simulink model "CEngDsT_DD"  (R2020b)
settings: configuration reference "cs_ert" (kept outside this file)
model workspace (MAT data in the model file):
  CEngDsT_DD_DT = 10
values from neighbouring files (symbols this model uses):
  CEngDsT_MaxCoolTemp = 150.0    [CEngDsT_DD.sldd]
  CEngDsT_MinCoolTemp = -50.0    [CEngDsT_DD.sldd]
  CEngDsT_tiMaxDefDeb_C = 200.0    [CEngDsT_DD.sldd]
  CEngDsT_tiMaxOKDeb_C = 200.0    [CEngDsT_DD.sldd]
  CEngDsT_tiMinDefDeb_C = 200.0    [CEngDsT_DD.sldd]
  CEngDsT_tiMinOKDeb_C = 200.0    [CEngDsT_DD.sldd]
  CEngDsT_tiPhysRngHiDefDeb_C = 200.0    [CEngDsT_DD.sldd]
  CEngDsT_tiPhysRngHiOKDeb_C = 200.0    [CEngDsT_DD.sldd]
  CEngDsT_tiPhysRngLoDefDeb_C = 200.0    [CEngDsT_DD.sldd]
  CEngDsT_tiPhysRngLoOKDeb_C = 200.0    [CEngDsT_DD.sldd]
  CEngDsT_tTransf_CUR : value not decoded    [CEngDsT_DD.sldd]
  CEngDsT_tTransf_CURX : value not decoded    [CEngDsT_DD.sldd]
  CEngDsT_uSRCMax_C = 5000.0    [CEngDsT_DD.sldd]
  CEngDsT_uSRCMin_C = 200.0    [CEngDsT_DD.sldd]
  FM_CEngDsT_SRC_FG_CA : value not decoded    [CEngDsT_DD.sldd]
libraries: sllib x5
settings Model: DataDictionary=CEngDsT_DD.sldd  EnableAccessToBaseWorkspace=off  Creator=zhoutinglin  LastModifiedBy=zhoutinglin
settings ConfigSetRef: SourceName=cs_ert

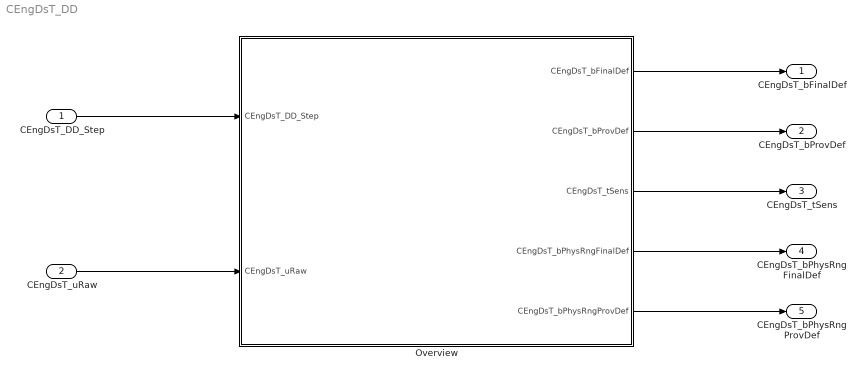
== system CEngDsT_DD ==
  CEngDsT_DD_Step : Inport  OutputFunctionCall=on
  CEngDsT_uRaw : Inport  Description=Raw ADC value of downstream engine coolant temperature sensor signal  Port=2  OutMin=0  OutMax=5000  OutDataTypeStr=Volt_mV2  Unit=mv  PortDimensions=[1 1]
  Overview : Subsystem
  CEngDsT_bFinalDef : Outport  Description=Status Sensor of the coolant temperature finally defect  OutMin=0  OutMax=1  OutDataTypeStr=boolean  PortDimensions=[1 1]
  CEngDsT_bProvDef : Outport  Description=Status Sensor of the coolant temperature temporary defect  Port=2  OutMin=0  OutMax=1  OutDataTypeStr=boolean  PortDimensions=[1 1]
  CEngDsT_tSens : Outport  Description=Sensed engine coolant temperature  Port=3  OutMin=-200  OutMax=200  OutDataTypeStr=Temp_C  Unit=deg  PortDimensions=[1 1]
  CEngDsT_bPhysRngFinalDef : Outport  Description=Status Sensor of the CEngDsT physical Signal range check finally defect  Port=4  OutMin=0  OutMax=1  OutDataTypeStr=boolean  PortDimensions=[1 1]
  CEngDsT_bPhysRngProvDef : Outport  Description=Status Sensor of the CEngDsT physical Signal range check temporary defect  Port=5  OutMin=0  OutMax=1  OutDataTypeStr=boolean  PortDimensions=[1 1]
  wires:
  Overview/4(CEngDsT_bPhysRngFinalDef) -> CEngDsT_bPhysRngFinalDef/1
  Overview/2(CEngDsT_bProvDef) -> CEngDsT_bProvDef/1
  Overview/1(CEngDsT_bFinalDef) -> CEngDsT_bFinalDef/1
  Overview/3(CEngDsT_tSens) -> CEngDsT_tSens/1
  Overview/5(CEngDsT_bPhysRngProvDef) -> CEngDsT_bPhysRngProvDef/1
  CEngDsT_uRaw/1 -> Overview/2(CEngDsT_uRaw)
  CEngDsT_DD_Step/1 -> Overview/1(CEngDsT_DD_Step)

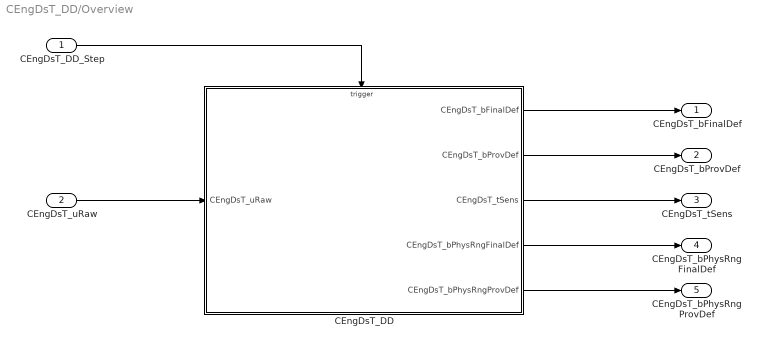
== system CEngDsT_DD/Overview ==
  CEngDsT_DD_Step : Inport
  CEngDsT_uRaw : Inport  Port=2
  CEngDsT_DD : Subsystem  RTWFcnName=CEngDsT_DDfun  RTWFileName=CEngDsT_DDfun
  CEngDsT_bFinalDef : Outport  VectorParamsAs1DForOutWhenUnconnected=off
  CEngDsT_bProvDef : Outport  Port=2  VectorParamsAs1DForOutWhenUnconnected=off
  CEngDsT_tSens : Outport  Port=3  VectorParamsAs1DForOutWhenUnconnected=off
  CEngDsT_bPhysRngFinalDef : Outport  Port=4  VectorParamsAs1DForOutWhenUnconnected=off
  CEngDsT_bPhysRngProvDef : Outport  Port=5  VectorParamsAs1DForOutWhenUnconnected=off
  wires:
  CEngDsT_uRaw/1 -> CEngDsT_DD/1(CEngDsT_uRaw)
  CEngDsT_DD/1(CEngDsT_bFinalDef) -> CEngDsT_bFinalDef/1
  CEngDsT_DD/2(CEngDsT_bProvDef) -> CEngDsT_bProvDef/1
  CEngDsT_DD/3(CEngDsT_tSens) -> CEngDsT_tSens/1
  CEngDsT_DD/4(CEngDsT_bPhysRngFinalDef) -> CEngDsT_bPhysRngFinalDef/1
  CEngDsT_DD/5(CEngDsT_bPhysRngProvDef) -> CEngDsT_bPhysRngProvDef/1
  CEngDsT_DD_Step/1 -> CEngDsT_DD/Trigger

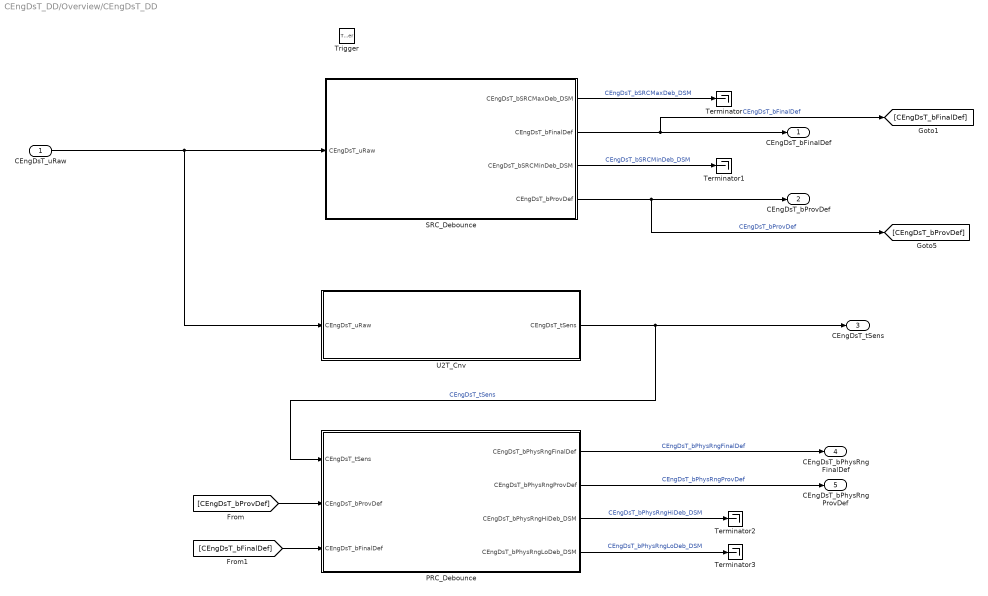
== system CEngDsT_DD/Overview/CEngDsT_DD ==
  CEngDsT_uRaw : Inport  Tag=mv
  Trigger : TriggerPort  TriggerType=function-call  VariantControl=Variant  PortDimensions=1
  PRC_Debounce : Subsystem
  SRC_Debounce : Subsystem
  Terminator{,1..3} (4 alike) : Terminator
  U2T_Cnv : Subsystem
  CEngDsT_bFinalDef : Outport  VectorParamsAs1DForOutWhenUnconnected=off
  CEngDsT_bProvDef : Outport  Port=2  VectorParamsAs1DForOutWhenUnconnected=off
  CEngDsT_tSens : Outport  Tag=deg  Port=3  VectorParamsAs1DForOutWhenUnconnected=off
  CEngDsT_bPhysRngFinalDef : Outport  Port=4  VectorParamsAs1DForOutWhenUnconnected=off
  CEngDsT_bPhysRngProvDef : Outport  Port=5  VectorParamsAs1DForOutWhenUnconnected=off
  wires:
  PRC_Debounce/3(CEngDsT_bPhysRngHiDeb_DSM) -> Terminator2/1  "CEngDsT_bPhysRngHiDeb_DSM"
  SRC_Debounce/3(CEngDsT_bSRCMinDeb_DSM) -> Terminator1/1  "CEngDsT_bSRCMinDeb_DSM"
  SRC_Debounce/1(CEngDsT_bSRCMaxDeb_DSM) -> Terminator/1  "CEngDsT_bSRCMaxDeb_DSM"
  [CEngDsT_bProvDef] -> PRC_Debounce/2(CEngDsT_bProvDef)
  PRC_Debounce/4(CEngDsT_bPhysRngLoDeb_DSM) -> Terminator3/1  "CEngDsT_bPhysRngLoDeb_DSM"
  [CEngDsT_bFinalDef] -> PRC_Debounce/3(CEngDsT_bFinalDef)
  CEngDsT_uRaw/1 -> U2T_Cnv/1(CEngDsT_uRaw), SRC_Debounce/1(CEngDsT_uRaw)
  PRC_Debounce/1(CEngDsT_bPhysRngFinalDef) -> CEngDsT_bPhysRngFinalDef/1  "CEngDsT_bPhysRngFinalDef"
  U2T_Cnv/1(CEngDsT_tSens) -> PRC_Debounce/1(CEngDsT_tSens), CEngDsT_tSens/1  "CEngDsT_tSens"
  SRC_Debounce/2(CEngDsT_bFinalDef) -> [CEngDsT_bFinalDef], CEngDsT_bFinalDef/1  "CEngDsT_bFinalDef"
  PRC_Debounce/2(CEngDsT_bPhysRngProvDef) -> CEngDsT_bPhysRngProvDef/1  "CEngDsT_bPhysRngProvDef"
  SRC_Debounce/4(CEngDsT_bProvDef) -> [CEngDsT_bProvDef], CEngDsT_bProvDef/1  "CEngDsT_bProvDef"

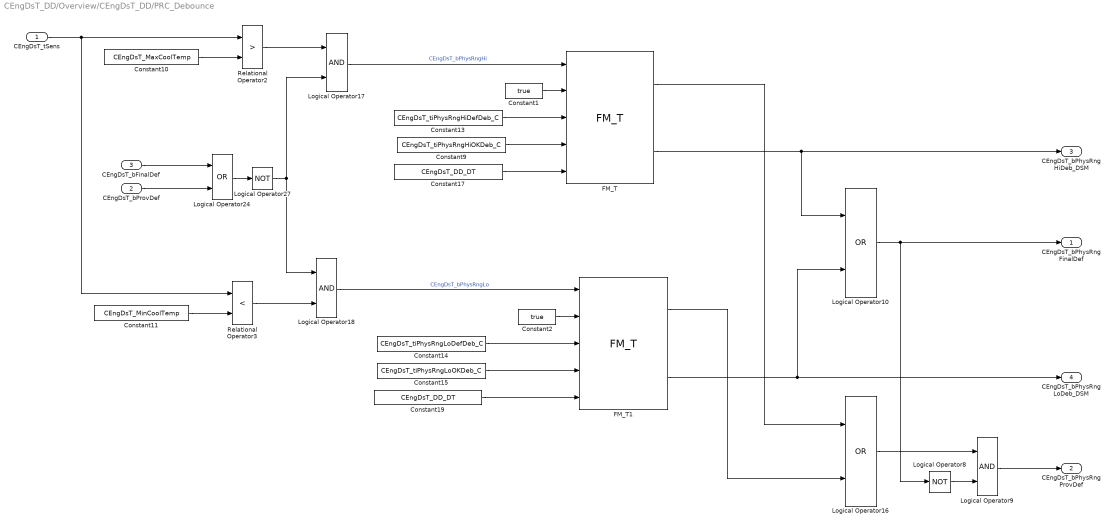
== system CEngDsT_DD/Overview/CEngDsT_DD/PRC_Debounce ==
  CEngDsT_tSens : Inport
  CEngDsT_bProvDef : Inport  Port=2
  CEngDsT_bFinalDef : Inport  Port=3
  Constant1 : Constant  Value=true  OutDataTypeStr=boolean
  Constant10 : Constant  Value=CEngDsT_MaxCoolTemp
  Constant11 : Constant  Value=CEngDsT_MinCoolTemp
  Constant13 : Constant  Value=CEngDsT_tiPhysRngHiDefDeb_C
  Constant14 : Constant  Value=CEngDsT_tiPhysRngLoDefDeb_C
  Constant15 : Constant  Value=CEngDsT_tiPhysRngLoOKDeb_C
  Constant17 : Constant  Value=CEngDsT_DD_DT  OutDataTypeStr=Inherit: Inherit via back propagation
  Constant19 : Constant  Value=CEngDsT_DD_DT  OutDataTypeStr=Inherit: Inherit via back propagation
  Constant2 : Constant  Value=true  OutDataTypeStr=boolean
  Constant9 : Constant  Value=CEngDsT_tiPhysRngHiOKDeb_C
  FM_T : sllib/Fault Manager/FM_T  Fault_ID=uint16(10)
      settings: AttributesFormatString=%<Fault_ID>  SourceProductName=sllib
  FM_T1 : sllib/Fault Manager/FM_T  Fault_ID=uint16(10)
      settings: AttributesFormatString=%<Fault_ID>  SourceProductName=sllib
  Logical Operator10 : Logic  Operator=OR  AllPortsSameDT=off  OutDataTypeStr=boolean
  Logical Operator16 : Logic  Operator=OR  AllPortsSameDT=off  OutDataTypeStr=boolean
  Logical Operator17 : Logic  AllPortsSameDT=off  OutDataTypeStr=boolean
  Logical Operator18 : Logic  AllPortsSameDT=off  OutDataTypeStr=boolean
  Logical Operator24 : Logic  Operator=OR  OutDataTypeStr=boolean
  Logical Operator27 : Logic  Operator=NOT  AllPortsSameDT=off  OutDataTypeStr=boolean
  Logical Operator8 : Logic  Operator=NOT  AllPortsSameDT=off  OutDataTypeStr=boolean
  Logical Operator9 : Logic  AllPortsSameDT=off  OutDataTypeStr=boolean
  Relational Operator2 : RelationalOperator  Operator=>  OutDataTypeStr=boolean  InputSameDT=on
  Relational Operator3 : RelationalOperator  Operator=<  OutDataTypeStr=boolean  RndMeth=Simplest  InputSameDT=on
  CEngDsT_bPhysRngFinalDef : Outport  Tag=-  VectorParamsAs1DForOutWhenUnconnected=off
  CEngDsT_bPhysRngProvDef : Outport  Tag=-  Port=2  VectorParamsAs1DForOutWhenUnconnected=off
  CEngDsT_bPhysRngHiDeb_DSM : Outport  Tag=-  Port=3  VectorParamsAs1DForOutWhenUnconnected=off
  CEngDsT_bPhysRngLoDeb_DSM : Outport  Tag=-  Port=4  VectorParamsAs1DForOutWhenUnconnected=off
  wires:
  CEngDsT_tSens/1 -> Relational Operator2/1, Relational Operator3/1
  Constant15/1 -> FM_T1/4
  Constant13/1 -> FM_T/3
  Constant9/1 -> FM_T/4
  Constant14/1 -> FM_T1/3
  Constant17/1 -> FM_T/5
  Constant19/1 -> FM_T1/5
  Constant10/1 -> Relational Operator2/2
  Logical Operator17/1 -> FM_T/1  "CEngDsT_bPhysRngHi"
  Constant11/1 -> Relational Operator3/2
  Logical Operator18/1 -> FM_T1/1  "CEngDsT_bPhysRngLo"
  FM_T/2 -> CEngDsT_bPhysRngHiDeb_DSM/1, Logical Operator10/1
  FM_T1/2 -> CEngDsT_bPhysRngLoDeb_DSM/1, Logical Operator10/2
  FM_T/1 -> Logical Operator16/1
  FM_T1/1 -> Logical Operator16/2
  Relational Operator2/1 -> Logical Operator17/1
  Logical Operator24/1 -> Logical Operator27/1
  Relational Operator3/1 -> Logical Operator18/2
  CEngDsT_bFinalDef/1 -> Logical Operator24/1
  CEngDsT_bProvDef/1 -> Logical Operator24/2
  Logical Operator27/1 -> Logical Operator17/2, Logical Operator18/1
  Logical Operator10/1 -> CEngDsT_bPhysRngFinalDef/1, Logical Operator8/1
  Logical Operator8/1 -> Logical Operator9/2
  Logical Operator9/1 -> CEngDsT_bPhysRngProvDef/1
  Constant1/1 -> FM_T/2
  Constant2/1 -> FM_T1/2
  Logical Operator16/1 -> Logical Operator9/1

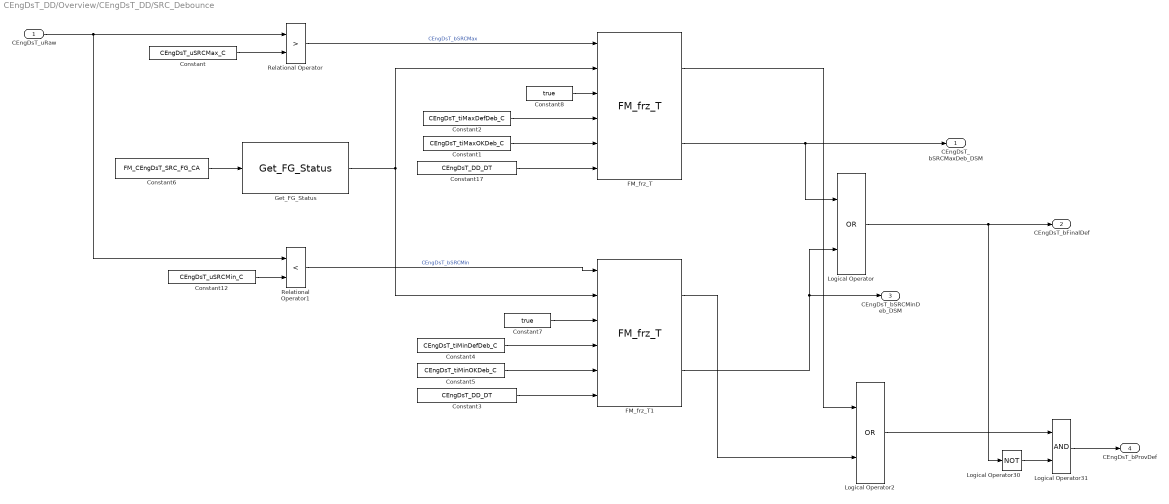
== system CEngDsT_DD/Overview/CEngDsT_DD/SRC_Debounce ==
  CEngDsT_uRaw : Inport  Tag=mv
  Constant : Constant  Value=CEngDsT_uSRCMax_C
  Constant1 : Constant  Value=CEngDsT_tiMaxOKDeb_C
  Constant12 : Constant  Value=CEngDsT_uSRCMin_C
  Constant17 : Constant  Value=CEngDsT_DD_DT  OutDataTypeStr=Inherit: Inherit via back propagation
  Constant2 : Constant  Value=CEngDsT_tiMaxDefDeb_C
  Constant3 : Constant  Value=CEngDsT_DD_DT  OutDataTypeStr=Inherit: Inherit via back propagation
  Constant4 : Constant  Value=CEngDsT_tiMinDefDeb_C
  Constant5 : Constant  Value=CEngDsT_tiMinOKDeb_C
  Constant6 : Constant  Value=FM_CEngDsT_SRC_FG_CA
  Constant7 : Constant  Value=true  OutDataTypeStr=boolean
  Constant8 : Constant  Value=true  OutDataTypeStr=boolean
  FM_frz_T : sllib/Fault Manager/FM_frz_T  Fault_ID=uint16(10)
      settings: AttributesFormatString=%<Fault_ID>  SourceProductName=sllib
  FM_frz_T1 : sllib/Fault Manager/FM_frz_T  Fault_ID=uint16(10)
      settings: AttributesFormatString=%<Fault_ID>  SourceProductName=sllib
  Get_FG_Status : sllib/Fault Manager/Get_FG_Status
      settings: SourceProductName=sllib
  Logical Operator : Logic  Operator=OR  AllPortsSameDT=off  OutDataTypeStr=boolean
  Logical Operator2 : Logic  Operator=OR  AllPortsSameDT=off  OutDataTypeStr=boolean
  Logical Operator30 : Logic  Operator=NOT  AllPortsSameDT=off  OutDataTypeStr=boolean
  Logical Operator31 : Logic  AllPortsSameDT=off  OutDataTypeStr=boolean
  Relational Operator : RelationalOperator  Operator=>  OutDataTypeStr=boolean  InputSameDT=on
  Relational Operator1 : RelationalOperator  Operator=<  OutDataTypeStr=boolean  InputSameDT=on
  CEngDsT_bSRCMaxDeb_DSM : Outport  Tag=-  VectorParamsAs1DForOutWhenUnconnected=off
  CEngDsT_bFinalDef : Outport  Tag=-  Port=2  VectorParamsAs1DForOutWhenUnconnected=off
  CEngDsT_bSRCMinDeb_DSM : Outport  Tag=-  Port=3  VectorParamsAs1DForOutWhenUnconnected=off
  CEngDsT_bProvDef : Outport  Tag=-  Port=4  VectorParamsAs1DForOutWhenUnconnected=off
  wires:
  CEngDsT_uRaw/1 -> Relational Operator1/1, Relational Operator/1
  Logical Operator/1 -> CEngDsT_bFinalDef/1, Logical Operator30/1
  Logical Operator30/1 -> Logical Operator31/2
  Logical Operator2/1 -> Logical Operator31/1
  Logical Operator31/1 -> CEngDsT_bProvDef/1
  Constant4/1 -> FM_frz_T1/4
  Constant1/1 -> FM_frz_T/5
  Constant2/1 -> FM_frz_T/4
  Constant5/1 -> FM_frz_T1/5
  Constant/1 -> Relational Operator/2
  Relational Operator/1 -> FM_frz_T/1  "CEngDsT_bSRCMax"
  Constant12/1 -> Relational Operator1/2
  Relational Operator1/1 -> FM_frz_T1/1  "CEngDsT_bSRCMin"
  FM_frz_T/2 -> Logical Operator/1, CEngDsT_bSRCMaxDeb_DSM/1
  FM_frz_T1/2 -> CEngDsT_bSRCMinDeb_DSM/1, Logical Operator/2
  Constant17/1 -> FM_frz_T/6
  Constant3/1 -> FM_frz_T1/6
  Constant6/1 -> Get_FG_Status/1
  Get_FG_Status/1 -> FM_frz_T1/2, FM_frz_T/2
  Constant7/1 -> FM_frz_T1/3
  Constant8/1 -> FM_frz_T/3
  FM_frz_T/1 -> Logical Operator2/1
  FM_frz_T1/1 -> Logical Operator2/2

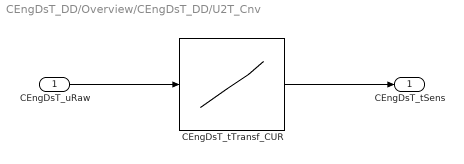
== system CEngDsT_DD/Overview/CEngDsT_DD/U2T_Cnv ==
  CEngDsT_uRaw : Inport  Tag=mv
  CEngDsT_tTransf_CUR : Lookup_n-D  DialogController=Simulink.DDGSource  NumberOfTableDimensions=1  BreakpointsForDimension1=CEngDsT_tTransf_CURX  BreakpointsForDimension2=CEngDsT_tTransf_CURX  BreakpointsForDimension1DataTypeStr=Inherit: Inherit from 'Breakpoint data'  IndexSearchMethod=Linear search  BeginIndexSearchUsingPreviousIndexResult=on  Table=CEngDsT_tTransf_CUR  TableDataTypeStr=Inherit: Inherit from 'Table data'  ExtrapMethod=Clip  RemoveProtectionInput=on  UseLastTableValue=on  InternalRulePriority=Speed  OutDataTypeStr=Inherit: Inherit from 'Table data'  SaturateOnIntegerOverflow=on
  CEngDsT_tSens : Outport  Tag=deg  VectorParamsAs1DForOutWhenUnconnected=off
  wires:
  CEngDsT_uRaw/1 -> CEngDsT_tTransf_CUR/1
  CEngDsT_tTransf_CUR/1 -> CEngDsT_tSens/1
